simulink model "MotorDriver_Sim_2020"  (R2020b)
settings: Solver=ode4  StartTime=0.0  StopTime=2  FixedStep=0.05  RelTol=1e-3
settings Model: Creator=005274  LastModifiedBy=005274

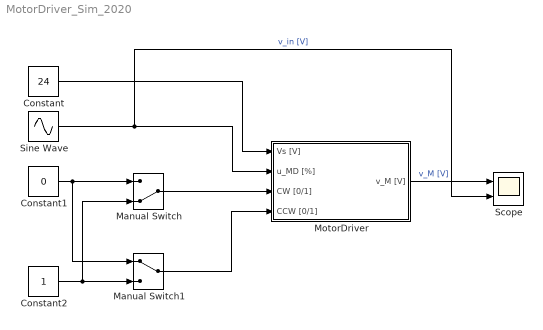
== system MotorDriver_Sim_2020 ==
  Constant : Constant  Value=24
  Constant1 : Constant  Value=0
  Constant2 : Constant
  Manual Switch : ManualSwitch  CurrentSetting=0
  Manual Switch1 : ManualSwitch
  MotorDriver : Subsystem  mask(MotorDriverModel){}
  Scope : Scope  NumInputPorts=2
  Sine Wave : Sin  Amplitude=50  Bias=50  Frequency=2*pi  SampleTime=0
  wires:
  Constant/1 -> MotorDriver/1(Vs [V])
  Sine Wave/1 -> MotorDriver/2(u_MD [%]), Scope/2  "v_in [V]"
  Constant2/1 -> Manual Switch/2, Manual Switch1/2
  Constant1/1 -> Manual Switch1/1, Manual Switch/1
  Manual Switch1/1 -> MotorDriver/4(CCW [0/1])
  Manual Switch/1 -> MotorDriver/3(CW [0/1])
  MotorDriver/1(v_M [V]) -> Scope/1  "v_M [V]"

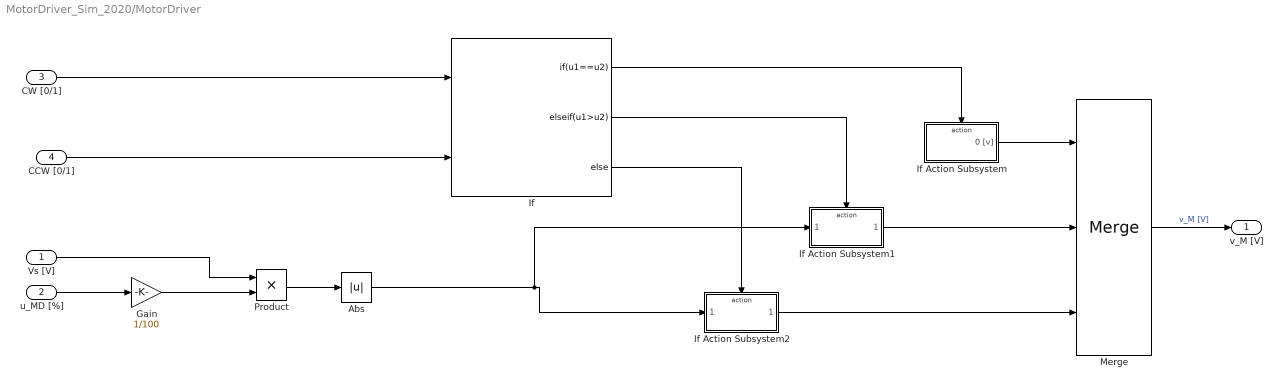
== system MotorDriver_Sim_2020/MotorDriver ==
  Vs [V] : Inport
  u_MD [%] : Inport  Port=2
  CW [0/1] : Inport  Port=3
  CCW [0/1] : Inport  Port=4
  Abs : Abs
  Gain : Gain  Gain=1/100
  If : If  NumInputs=2  IfExpression=u1==u2  ElseIfExpressions=u1>u2
  If Action Subsystem : Subsystem  TreatAsAtomicUnit=on
  If Action Subsystem1 : Subsystem  TreatAsAtomicUnit=on
  If Action Subsystem2 : Subsystem  TreatAsAtomicUnit=on
  Merge : Merge  Inputs=3
  Product : Product
  v_M [V] : Outport
  wires:
  Product/1 -> Abs/1
  Gain/1 -> Product/2
  If Action Subsystem1/1(v_M [V]) -> Merge/2
  If Action Subsystem2/1(-v_M [V]) -> Merge/3
  If/2 -> If Action Subsystem1/Action
  Merge/1 -> v_M [V]/1  "v_M [V]"
  If Action Subsystem/1(0 [v]) -> Merge/1
  If/1 -> If Action Subsystem/Action
  Vs [V]/1 -> Product/1
  If/3 -> If Action Subsystem2/Action
  u_MD [%]/1 -> Gain/1
  Abs/1 -> If Action Subsystem1/1(|v_M| [V]), If Action Subsystem2/1(|v_M| [V])
  CW [0/1]/1 -> If/1
  CCW [0/1]/1 -> If/2

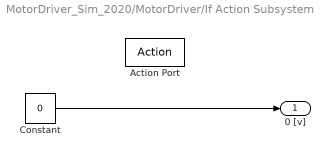
== system MotorDriver_Sim_2020/MotorDriver/If Action Subsystem ==
  Action Port : ActionPort  ActionPortLabel=if(u1==u2)
  Constant : Constant  Value=0
  0 [v] : Outport
  wires:
  Constant/1 -> 0 [v]/1

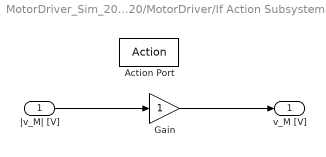
== system MotorDriver_Sim_2020/MotorDriver/If Action Subsystem1 ==
  |v_M| [V] : Inport
  Action Port : ActionPort  ActionPortLabel=elseif(u1>u2)
  Gain : Gain
  v_M [V] : Outport
  wires:
  |v_M| [V]/1 -> Gain/1
  Gain/1 -> v_M [V]/1

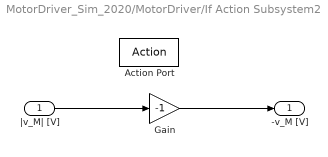
== system MotorDriver_Sim_2020/MotorDriver/If Action Subsystem2 ==
  |v_M| [V] : Inport
  Action Port : ActionPort  ActionPortLabel=else
  Gain : Gain  Gain=-1
  -v_M [V] : Outport
  wires:
  |v_M| [V]/1 -> Gain/1
  Gain/1 -> -v_M [V]/1
